simulink model "SF051A_SnsrOffsLrng"  (R2013b)
settings: Solver=FixedStepDiscrete  SolverMode=SingleTasking  StartTime=0.0  StopTime=1  FixedStep=0.002  RelTol=1e-3
undefined symbols (not defined in the file): ARCHGLBPRM_10MILLISEC_SEC_F32, ARCHGLBPRM_2MILLISEC_SEC_F32, ARCHGLBPRM_2PI_ULS_F32, ARCHGLBPRM_FLOATZEROTHD_ULS_F32, ARCHGLBPRM_PIOVER180_ULS_F32, CNV100MICROSECTOMILLISEC_MILLISECPERCNT_F32, CNV100MICROSECTOSEC_SECPERCNT_F32, COVRAMTRXNIT_ULS_F32, HWAUTHYTHD_ULS_F32, HWTQLRNGSTSLRND_CNT_U08, HWTQLRNGSTSNEGOFFS_CNT_U08, HWTQLRNGSTSNOTLRND_CNT_U08, HWTQLRNGSTSPOSOFFS_CNT_U08, HWTQLRNGSTSZEROOFFS_CNT_U08, HWTQLRNGTMRHILIM_SEC_F32, IDYMTRX_ULS_F32, IVS10MS_ULSPERSEC_F32, LRNGFILTICON_ULS_F32, NvmGetErrSts1, ONE_ULS_F32, SnsrOffsLrnd, SnsrOffsLrngFctEna, SnsrOffsLrngHwAgLrngDrvgDstThd, SnsrOffsLrngHwAgLrngEna, SnsrOffsLrngHwAgLrngHwVelThd, SnsrOffsLrngHwAgLrngSysTqThd, SnsrOffsLrngHwAgLrngSysTqThdMed, SnsrOffsLrngHwAgLrngSysTqThdTrustd, SnsrOffsLrngHwAgLrngSysTqThdWide, SnsrOffsLrngHwAgLrngTi, SnsrOffsLrngHwAgLrngVehSpdThd, SnsrOffsLrngHwAgLrngYawOffsDbnd, SnsrOffsLrngHwAgLrngYawRateThd, SnsrOffsLrngHwAgOffsLim, SnsrOffsLrngHwTqLrngEna, SnsrOffsLrngHwTqLrngEnaTiThd, SnsrOffsLrngHwTqLrngHwAgDbnd, SnsrOffsLrngHwTqLrngHwAgThd, SnsrOffsLrngHwTqLrngHwTqThd, SnsrOffsLrngHwTqLrngHwTqZeroOffsThd, SnsrOffsLrngHwTqLrngHwVelThd, SnsrOffsLrngHwTqLrngMeasTi, SnsrOffsLrngHwTqLrngMeasTiScar, SnsrOffsLrngHwTqLrngSampleImbThd1, SnsrOffsLrngHwTqLrngSampleImbThd2, SnsrOffsLrngHwTqLrngSampleThd1, SnsrOffsLrngHwTqLrngSampleThd2, SnsrOffsLrngHwTqLrngTiWghtCoeff, SnsrOffsLrngHwTqLrngVehSpdThd, SnsrOffsLrngHwTqOffsLim, SnsrOffsLrngSampleCntForHwTqLrngRst, SnsrOffsLrngTqInpDetnPwrEstimnThd, SnsrOffsLrngTqInpDetnSinGenrAmp, SnsrOffsLrngTqInpDetnSinGenrFrq, SnsrOffsLrngTqInpDetnStg1FilGain, SnsrOffsLrngTqInpDetnStg1WinSize, SnsrOffsLrngTqInpDetnStg2FilGainCen, SnsrOffsLrngTqInpDetnStg2FilGainDwn, SnsrOffsLrngTqInpDetnStg2FilGainUp, SnsrOffsLrngTqInpDetnStg2WinSize ... (+15)
libraries: Fil x34, FixdToFloat x17, FloatToFixd x16, NxtrLim x15, simulink x12, NxtrAbslt x12, NxtrNvM x8, NxtrMin x5, NxtrMath x3
(part 2 of 11)

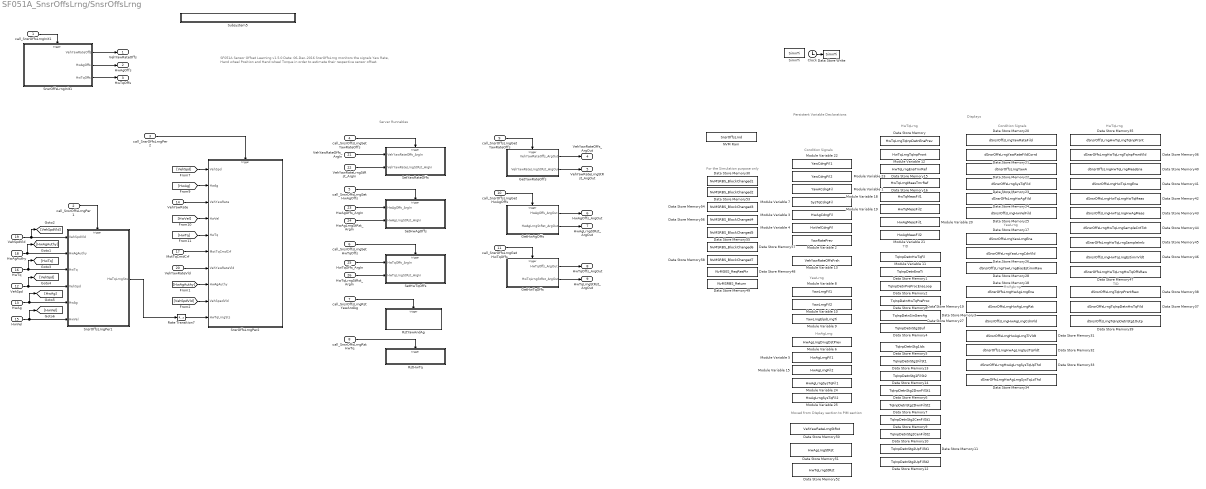
== system SF051A_SnsrOffsLrng/SnsrOffsLrng ==
  note: Moved from DIsplay section to PIM section
  note: For the Simulation purpose only
  note: TID
  note: TID
  note: Condition Signals
  note: Server Runnables
  note: Persistent Variable Declarations
  note: Displays
  note: YawLrng
  note: HwAgLrng
  note: HwTqLrng
  note: Condition Signals
  note: YawLrng
  note: HwAgLrng
  note: HwTqLrng
  note: SF051A  Sensor Offset Learning
      | v1.5.0 	Date: 06-Dec-2016
      |
      | SnsrOffsLrng monitors the signals Yaw Rate, Hand wheel Position and Hand wheel Torque in order to estimate their respective sensor offset.
  call_SnsrOffsLrngInit1 : Inport  RequirementInfo={'linktype_rmi_doors' '0000babd (/E-STEER Core/SubSystem Specifications/Application Functions/SF051A Sensor Offset Learning)' '#SF051A_46' 'true' 'REQ:SF051A_46' '' ; 'linktype_rmi_doors' '0000babd (/E-STEER Core/SubSystem Specifications/Application Functions/SF051A Sensor Offset Learning)' '#SF051A_210' 'true' 'REQ:SF051A_210' '' } %GIDa_b5548396_b826_4291_b305_596c7c623535
  call_SnsrOffsLrngPer1 : Inport  RequirementInfo={'linktype_rmi_doors' '0000babd (/E-STEER Core/SubSystem Specifications/Application Functions/SF051A Sensor Offset Learning)' '#SF051A_207' 'true' 'REQ:SF051A_207' '' } %GIDa_b76faf1e_0a38_4892_bc53_8cf50d1431b9  Port=2
  call_SnsrOffsLrngPer2 : Inport  RequirementInfo={'linktype_rmi_doors' '0000babd (/E-STEER Core/SubSystem Specifications/Application Functions/SF051A Sensor Offset Learning)' '#SF051A_206' 'true' 'REQ:SF051A_206' '' ; 'linktype_rmi_doors' '0000babd (/E-STEER Core/SubSystem Specifications/Application Functions/SF051A Sensor Offset Learning)' '#SF051A_208' 'true' 'REQ:SF051A_208' '' } %GIDa_53f91c8f_8084_4b7b_a29a_1f5e6264ef74  Port=3
  call_SnsrOffsLrngSetYawRateOffs : Inport  RequirementInfo={'linktype_rmi_doors' '0000babd (/E-STEER Core/SubSystem Specifications/Application Functions/SF051A Sensor Offset Learning)' '#SF051A_58' 'true' 'REQ:SF051A_58' '' ; 'linktype_rmi_doors' '0000babd (/E-STEER Core/SubSystem Specifications/Application Functions/SF051A Sensor Offset Learning)' '#SF051A_237' 'true' 'REQ:SF051A_237' '' } %GIDa_9ebfcf6d_e478_413c_8c0c_a98fbe6df9d3  Port=4
  call_SnsrOffsLrngSetHwAgOffs : Inport  RequirementInfo={'linktype_rmi_doors' '0000babd (/E-STEER Core/SubSystem Specifications/Application Functions/SF051A Sensor Offset Learning)' '#SF051A_215' 'true' 'REQ:SF051A_215' '' ; 'linktype_rmi_doors' '0000babd (/E-STEER Core/SubSystem Specifications/Application Functions/SF051A Sensor Offset Learning)' '#SF051A_236' 'true' 'REQ:SF051A_236' '' } %GIDa_c1056425_e33c_42d4_9d68_7c8d70d8efa0  Port=5
  call_SnsrOffsLrngSetHwTqOffs : Inport  RequirementInfo={'linktype_rmi_doors' '0000babd (/E-STEER Core/SubSystem Specifications/Application Functions/SF051A Sensor Offset Learning)' '#SF051A_213' 'true' 'REQ:SF051A_213' '' ; 'linktype_rmi_doors' '0000babd (/E-STEER Core/SubSystem Specifications/Application Functions/SF051A Sensor Offset Learning)' '#SF051A_238' 'true' 'REQ:SF051A_238' '' } %GIDa_875b11dc_9366_4bb8_a936_d7d6b5c30bfa  Port=6
  call_SnsrOffsLrngRstYawAndAg : Inport  RequirementInfo={'linktype_rmi_doors' '0000babd (/E-STEER Core/SubSystem Specifications/Application Functions/SF051A Sensor Offset Learning)' '#SF051A_211' 'true' 'REQ:SF051A_211' '' ; 'linktype_rmi_doors' '0000babd (/E-STEER Core/SubSystem Specifications/Application Functions/SF051A Sensor Offset Learning)' '#SF051A_234' 'true' 'REQ:SF051A_234' '' } %GIDa_4fb6cb0e_ae58_45eb_a23a_8ef4f0284ae6  Port=7
  call_SnsrOffsLrngRstHwTq : Inport  RequirementInfo={'linktype_rmi_doors' '0000babd (/E-STEER Core/SubSystem Specifications/Application Functions/SF051A Sensor Offset Learning)' '#SF051A_216' 'true' 'REQ:SF051A_216' '' ; 'linktype_rmi_doors' '0000babd (/E-STEER Core/SubSystem Specifications/Application Functions/SF051A Sensor Offset Learning)' '#SF051A_235' 'true' 'REQ:SF051A_235' '' } %GIDa_99803fa3_df4f_4cf4_914f_3ed5b7add009  Port=8
  call_SnsrOffsLrngGetYawRateOffs : Inport  RequirementInfo={'linktype_rmi_doors' '0000babd (/E-STEER Core/SubSystem Specifications/Application Functions/SF051A Sensor Offset Learning)' '#SF051A_217' 'true' 'REQ:SF051A_217' '' ; 'linktype_rmi_doors' '0000babd (/E-STEER Core/SubSystem Specifications/Application Functions/SF051A Sensor Offset Learning)' '#SF051A_229' 'true' 'REQ:SF051A_229' '' } %GIDa_2fe70a0d_0969_4657_91b9_882eb0d6e8f3  Port=9
  call_SnsrOffsLrngGetHwAgOffs : Inport  RequirementInfo={'linktype_rmi_doors' '0000babd (/E-STEER Core/SubSystem Specifications/Application Functions/SF051A Sensor Offset Learning)' '#SF051A_214' 'true' 'REQ:SF051A_214' '' ; 'linktype_rmi_doors' '0000babd (/E-STEER Core/SubSystem Specifications/Application Functions/SF051A Sensor Offset Learning)' '#SF051A_231' 'true' 'REQ:SF051A_231' '' } %GIDa_e15fe6be_8261_450e_92cb_69dfcf136740  Port=10
  call_SnsrOffsLrngGetHwTqOffs : Inport  RequirementInfo={'linktype_rmi_doors' '0000babd (/E-STEER Core/SubSystem Specifications/Application Functions/SF051A Sensor Offset Learning)' '#SF051A_212' 'true' 'REQ:SF051A_212' '' ; 'linktype_rmi_doors' '0000babd (/E-STEER Core/SubSystem Specifications/Application Functions/SF051A Sensor Offset Learning)' '#SF051A_233' 'true' 'REQ:SF051A_233' '' } %GIDa_11a16519_835e_433c_aee1_e13e931b852c  Port=11
  VehSpd : Inport  RequirementInfo={'linktype_rmi_doors' '0000babd (/E-STEER Core/SubSystem Specifications/Application Functions/SF051A Sensor Offset Learning)' '#SF051A_73' 'true' 'REQ:SF051A_73' '' } %GIDa_6cab4be4_5aaa_4f06_92e7_199f0ab886cf  Port=12
  HwAg : Inport  RequirementInfo={'linktype_rmi_doors' '0000babd (/E-STEER Core/SubSystem Specifications/Application Functions/SF051A Sensor Offset Learning)' '#SF051A_71' 'true' 'REQ:SF051A_71' '' } %GIDa_43d75a5a_0460_4bf8_8d04_3cab9ef42970  Port=13
  VehYawRate : Inport  RequirementInfo={'linktype_rmi_doors' '0000babd (/E-STEER Core/SubSystem Specifications/Application Functions/SF051A Sensor Offset Learning)' '#SF051A_74' 'true' 'REQ:SF051A_74' '' } %GIDa_85702be3_759d_431f_afdd_1834d4451958  Port=14
  HwVel : Inport  RequirementInfo={'linktype_rmi_doors' '0000babd (/E-STEER Core/SubSystem Specifications/Application Functions/SF051A Sensor Offset Learning)' '#SF051A_76' 'true' 'REQ:SF051A_76' '' } %GIDa_aea7e932_9aba_450e_a5e8_854429f45d9e  Port=15
  HwTq : Inport  RequirementInfo={'linktype_rmi_doors' '0000babd (/E-STEER Core/SubSystem Specifications/Application Functions/SF051A Sensor Offset Learning)' '#SF051A_12' 'true' 'REQ:SF051A_12' '' } %GIDa_419a1852_02b0_4166_858b_b9defd51bcfd  Port=16
  MotTqCmdCrf : Inport  RequirementInfo={'linktype_rmi_doors' '0000babd (/E-STEER Core/SubSystem Specifications/Application Functions/SF051A Sensor Offset Learning)' '#SF051A_78' 'true' 'REQ:SF051A_78' '' } %GIDa_8d4508d2_1c4e_4f52_beaa_b504c4c90863  Port=17
  HwAgAuthy : Inport  RequirementInfo={'linktype_rmi_doors' '0000babd (/E-STEER Core/SubSystem Specifications/Application Functions/SF051A Sensor Offset Learning)' '#SF051A_75' 'true' 'REQ:SF051A_75' '' } %GIDa_db428556_ad0a_4a7e_ac2f_05533f125a8d  Port=18
  VehSpdVld : Inport  RequirementInfo={'linktype_rmi_doors' '0000babd (/E-STEER Core/SubSystem Specifications/Application Functions/SF051A Sensor Offset Learning)' '#SF051A_72' 'true' 'REQ:SF051A_72' '' } %GIDa_549d97e8_51ee_4f7d_a4b4_1f4d4fa29ac3  Port=19
  VehYawRateVld : Inport  RequirementInfo={'linktype_rmi_doors' '0000babd (/E-STEER Core/SubSystem Specifications/Application Functions/SF051A Sensor Offset Learning)' '#SF051A_77' 'true' 'REQ:SF051A_77' '' } %GIDa_9dcd395b_e912_4846_98d8_9746842c61cb  Port=20
  VehYawRateOffs_ArgIn : Inport  RequirementInfo={'linktype_rmi_doors' '0000babd (/E-STEER Core/SubSystem Specifications/Application Functions/SF051A Sensor Offset Learning)' '#SF051A_58' 'true' 'REQ:SF051A_58' '' } %GIDa_f87127ae_4fd6_4799_a67b_96b70cf59f57  Port=21
  VehYawRateLrngStRst_ArgIn : Inport  RequirementInfo={'linktype_rmi_doors' '0000babd (/E-STEER Core/SubSystem Specifications/Application Functions/SF051A Sensor Offset Learning)' '#SF051A_237' 'true' 'REQ:SF051A_237' '' } %GIDa_de74ad38_9d1d_42b4_98c9_5d5518144ab9  Port=22
  HwAgOffs_ArgIn : Inport  RequirementInfo={'linktype_rmi_doors' '0000babd (/E-STEER Core/SubSystem Specifications/Application Functions/SF051A Sensor Offset Learning)' '#SF051A_215' 'true' 'REQ:SF051A_215' '' } %GIDa_6970447d_a6e4_4a38_8aa3_8925f782d5d0  Port=23
  HwAgLrngStRst_ArgIn : Inport  RequirementInfo={'linktype_rmi_doors' '0000babd (/E-STEER Core/SubSystem Specifications/Application Functions/SF051A Sensor Offset Learning)' '#SF051A_236' 'true' 'REQ:SF051A_236' '' } %GIDa_7c9b4228_d04e_41fe_8d4c_bf60f37f9eec  Port=24
  HwTqOffs_ArgIn : Inport  RequirementInfo={'linktype_rmi_doors' '0000babd (/E-STEER Core/SubSystem Specifications/Application Functions/SF051A Sensor Offset Learning)' '#SF051A_213' 'true' 'REQ:SF051A_213' '' } %GIDa_303f314c_88b6_4fa0_bca5_4af63bedbea5  Port=25
  HwTqLrngStRst_ArgIn : Inport  RequirementInfo={'linktype_rmi_doors' '0000babd (/E-STEER Core/SubSystem Specifications/Application Functions/SF051A Sensor Offset Learning)' '#SF051A_238' 'true' 'REQ:SF051A_238' '' } %GIDa_34ca438f_6084_484d_a532_1ca155d267e9  Port=26
  Clock : Clock
  Data Store Memory : DataStoreMemory  DataStoreName=HwTqLrngTqInpDetnEnaPrev  OutDataTypeStr=boolean  StateMustResolveToSignalObject=on
  Data Store Memory1 : DataStoreMemory  DataStoreName=TqInpDetnEnaTi  StateMustResolveToSignalObject=on
  Data Store Memory10 : DataStoreMemory  DataStoreName=TqInpDetnStg2CenFilSt2  StateMustResolveToSignalObject=on
  Data Store Memory11 : DataStoreMemory  DataStoreName=TqInpDetnStg2UpFilSt1  StateMustResolveToSignalObject=on
  Data Store Memory12 : DataStoreMemory  DataStoreName=TqInpDetnStg2UpFilSt2  StateMustResolveToSignalObject=on
  Data Store Memory13 : DataStoreMemory  DataStoreName=TqInpDetnStg1FilSt1  StateMustResolveToSignalObject=on
  Data Store Memory14 : DataStoreMemory  DataStoreName=TqInpDetnStg1FilSt2  StateMustResolveToSignalObject=on
  Data Store Memory15 : DataStoreMemory  DataStoreName=HwTqLrngEnaTmrRef  StateMustResolveToSignalObject=on
  Data Store Memory16 : DataStoreMemory  DataStoreName=HwTqLrngMeasTmrRef  OutDataTypeStr=uint32  StateMustResolveToSignalObject=on
  Data Store Memory17 : DataStoreMemory  DataStoreName=dSnsrOffsLrngYawLrngEna  StateMustResolveToSignalObject=on
  Data Store Memory18 : DataStoreMemory  DataStoreName=dSnsrOffsLrngHwAgLrngEna  StateMustResolveToSignalObject=on
  Data Store Memory19 : DataStoreMemory  DataStoreName=dSnsrOffsLrngHwAgLrngRst  StateMustResolveToSignalObject=on
  Data Store Memory2 : DataStoreMemory  DataStoreName=TqInpDetnPreProcEnaLoop  OutDataTypeStr=uint16  StateMustResolveToSignalObject=on
  Data Store Memory20 : DataStoreMemory  DataStoreName=dSnsrOffsLrngYawRateFild  StateMustResolveToSignalObject=on
  Data Store Memory21 : DataStoreMemory  DataStoreName=dSnsrOffsLrngYawRateFildCorrd  StateMustResolveToSignalObject=on
  Data Store Memory22 : DataStoreMemory  DataStoreName=dSnsrOffsLrngYawA  StateMustResolveToSignalObject=on
  Data Store Memory23 : DataStoreMemory  DataStoreName=dSnsrOffsLrngSysTqFild  StateMustResolveToSignalObject=on
  Data Store Memory24 : DataStoreMemory  DataStoreName=dSnsrOffsLrngHwAgFild  StateMustResolveToSignalObject=on
  Data Store Memory25 : DataStoreMemory  DataStoreName=dSnsrOffsLrngHwVelFild  StateMustResolveToSignalObject=on
  Data Store Memory26 : DataStoreMemory  DataStoreName=dSnsrOffsLrngYawLrngCdnVld  StateMustResolveToSignalObject=on
  Data Store Memory27 : DataStoreMemory  DataStoreName=dSnsrOffsLrngHwAgLrngCdnVld  StateMustResolveToSignalObject=on
  Data Store Memory28 : DataStoreMemory  DataStoreName=dSnsrOffsLrngYawLrngBiasEstimnRaw  StateMustResolveToSignalObject=on
  Data Store Memory3 : DataStoreMemory  DataStoreName=TqInpDetnSinGenrAg  StateMustResolveToSignalObject=on
  Data Store Memory30 : DataStoreMemory  DataStoreName=NvMSRBS_BlockChanged1
  Data Store Memory31 : DataStoreMemory  DataStoreName=dSnsrOffsLrngHwAgLrngTiVldt  StateMustResolveToSignalObject=on
  Data Store Memory32 : DataStoreMemory  DataStoreName=dSnsrOffsLrngHwAgLrngSysTqVldt  StateMustResolveToSignalObject=on
  Data Store Memory33 : DataStoreMemory  DataStoreName=dSnsrOffsLrngHwAgLrngSysTqUpThd  StateMustResolveToSignalObject=on
  Data Store Memory34 : DataStoreMemory  DataStoreName=dSnsrOffsLrngHwAgLrngSysTqLoThd  StateMustResolveToSignalObject=on
  Data Store Memory35 : DataStoreMemory  DataStoreName=dSnsrOffsLrngHwTqLrngTqInpPrsnt  StateMustResolveToSignalObject=on
  Data Store Memory36 : DataStoreMemory  DataStoreName=dSnsrOffsLrngHwTqLrngTqInpPrsntVld  StateMustResolveToSignalObject=on
  Data Store Memory37 : DataStoreMemory  DataStoreName=dSnsrOffsLrngTqInpDetnHwTqFild  StateMustResolveToSignalObject=on
  Data Store Memory38 : DataStoreMemory  DataStoreName=dSnsrOffsLrngTqInpPrsntRaw  StateMustResolveToSignalObject=on
  Data Store Memory39 : DataStoreMemory  DataStoreName=dSnsrOffsLrngTqInpDetnStg1Outp  StateMustResolveToSignalObject=on
  Data Store Memory4 : DataStoreMemory  DataStoreName=TqInpDetnStg1Buf  InitialValue=[]  StateMustResolveToSignalObject=on
      settings: AttributesFormatString=Initialize as array of 72 zeros because buffer size cal = 1 to 72.
  Data Store Memory40 : DataStoreMemory  DataStoreName=dSnsrOffsLrngHwTqLrngMeasEna  StateMustResolveToSignalObject=on
  Data Store Memory41 : DataStoreMemory  DataStoreName=dSnsrOffsLrngHwTqLrngEna  StateMustResolveToSignalObject=on
  Data Store Memory42 : DataStoreMemory  DataStoreName=dSnsrOffsLrngHwTqLrngHwTqMeas  StateMustResolveToSignalObject=on
  Data Store Memory43 : DataStoreMemory  DataStoreName=dSnsrOffsLrngHwTqLrngHwAgMeas  StateMustResolveToSignalObject=on
  Data Store Memory44 : DataStoreMemory  DataStoreName=dSnsrOffsLrngHwTqLrngSampleCntTot  StateMustResolveToSignalObject=on
  Data Store Memory45 : DataStoreMemory  DataStoreName=dSnsrOffsLrngHwTqLrngSampleImb  StateMustResolveToSignalObject=on
  Data Store Memory46 : DataStoreMemory  DataStoreName=dSnsrOffsLrngHwTqLrngEstimnVldt  StateMustResolveToSignalObject=on
  Data Store Memory47 : DataStoreMemory  DataStoreName=dSnsrOffsLrngHwTqLrngHwTqOffsRaw  StateMustResolveToSignalObject=on
  Data Store Memory48 : DataStoreMemory  DataStoreName=NvMGES_ReqResPtr  InitialValue=NvmGetErrSts1.REQUEST_NOT_OK  OutDataTypeStr=Enum: NvmGetErrSts1
  Data Store Memory49 : DataStoreMemory  DataStoreName=NvMSRBS_Return
  Data Store Memory5 : DataStoreMemory  DataStoreName=TqInpDetnStg1Idx  StateMustResolveToSignalObject=on
  Data Store Memory50 : DataStoreMemory  DataStoreName=VehYawRateLrngStRst  StateMustResolveToSignalObject=on
  Data Store Memory51 : DataStoreMemory  DataStoreName=HwAgLrngStRst  StateMustResolveToSignalObject=on
  Data Store Memory52 : DataStoreMemory  DataStoreName=HwTqLrngStRst  StateMustResolveToSignalObject=on
  Data Store Memory53 : DataStoreMemory  DataStoreName=NvMSRBS_BlockChanged2
  Data Store Memory54 : DataStoreMemory  DataStoreName=NvMSRBS_BlockChanged3
  Data Store Memory55 : DataStoreMemory  DataStoreName=NvMSRBS_BlockChanged5
  Data Store Memory56 : DataStoreMemory  DataStoreName=NvMSRBS_BlockChanged4
  Data Store Memory57 : DataStoreMemory  DataStoreName=NvMSRBS_BlockChanged6
  Data Store Memory58 : DataStoreMemory  DataStoreName=NvMSRBS_BlockChanged7
  Data Store Memory6 : DataStoreMemory  DataStoreName=TqInpDetnStg2DwnFilSt1  StateMustResolveToSignalObject=on
  Data Store Memory7 : DataStoreMemory  DataStoreName=TqInpDetnStg2DwnFilSt2  StateMustResolveToSignalObject=on
  Data Store Memory8 : DataStoreMemory  DataStoreName=TqInpDetnHwTqPreProc  StateMustResolveToSignalObject=on
  Data Store Memory9 : DataStoreMemory  DataStoreName=TqInpDetnStg2CenFilSt1  StateMustResolveToSignalObject=on
  Data Store Write : DataStoreWrite  DataStoreName=SimnTi
  GetHwAgOffs : Subsystem  RequirementInfo={'linktype_rmi_doors' '0000babd (/E-STEER Core/SubSystem Specifications/Application Functions/SF051A Sensor Offset Learning)' '#SF051A_214' 'true' 'REQ:SF051A_214' '' ; 'linktype_rmi_doors' '0000babd (/E-STEER Core/SubSystem Specifications/Application Functions/SF051A Sensor Offset Learning)' '#SF051A_231' 'true' 'REQ:SF051A_231' '' } %GIDa_829ee463_2f90_4434_8814_18ee114c17a8  TreatAsAtomicUnit=on
  GetHwTqOffs : Subsystem  RequirementInfo={'linktype_rmi_doors' '0000babd (/E-STEER Core/SubSystem Specifications/Application Functions/SF051A Sensor Offset Learning)' '#SF051A_212' 'true' 'REQ:SF051A_212' '' ; 'linktype_rmi_doors' '0000babd (/E-STEER Core/SubSystem Specifications/Application Functions/SF051A Sensor Offset Learning)' '#SF051A_233' 'true' 'REQ:SF051A_233' '' } %GIDa_f3af8530_8b46_4cec_b6bb_ea1c7cec3483  TreatAsAtomicUnit=on
  GetYawRateOffs : Subsystem  RequirementInfo={'linktype_rmi_doors' '0000babd (/E-STEER Core/SubSystem Specifications/Application Functions/SF051A Sensor Offset Learning)' '#SF051A_217' 'true' 'REQ:SF051A_217' '' ; 'linktype_rmi_doors' '0000babd (/E-STEER Core/SubSystem Specifications/Application Functions/SF051A Sensor Offset Learning)' '#SF051A_229' 'true' 'REQ:SF051A_229' '' } %GIDa_bc715bf0_598f_44bb_a83a_ee16c1cb044c  TreatAsAtomicUnit=on
  Module Variable 1 : DataStoreMemory  DataStoreName=YawACdngFil  InitialValue=struct('FilSt',single(0),'FilGain',single(0))  StateMustResolveToSignalObject=on
  Module Variable 10 : DataStoreMemory  DataStoreName=YawLrngFil2  InitialValue=struct('FilSt',single(0),'FilGain',single(0))  StateMustResolveToSignalObject=on
  Module Variable 11 : DataStoreMemory  DataStoreName=TqInpDetnHwTqFil  InitialValue=struct('FilSt',single(0),'FilGain',single(0))  StateMustResolveToSignalObject=on
  Module Variable 12 : DataStoreMemory  DataStoreName=HwTqLrngTqInpPrsnt  OutDataTypeStr=boolean  StateMustResolveToSignalObject=on
  Module Variable 13 : DataStoreMemory  DataStoreName=VehYawRateOffsFrsh  StateMustResolveToSignalObject=on
  Module Variable 15 : DataStoreMemory  DataStoreName=HwAgLrngFil2  InitialValue=struct('FilSt',single(0),'FilGain',single(0))  StateMustResolveToSignalObject=on
  Module Variable 18 : DataStoreMemory  DataStoreName=HwTqMeasFil1  InitialValue=struct('FilSt',single(0),'FilGain',single(0))  StateMustResolveToSignalObject=on
  Module Variable 19 : DataStoreMemory  DataStoreName=HwTqMeasFil2  InitialValue=struct('FilSt',single(0),'FilGain',single(0))  StateMustResolveToSignalObject=on
  Module Variable 2 : DataStoreMemory  DataStoreName=YawRatePrev  StateMustResolveToSignalObject=on
  Module Variable 20 : DataStoreMemory  DataStoreName=HwAgMeasFil1  InitialValue=struct('FilSt',single(0),'FilGain',single(0))  StateMustResolveToSignalObject=on
  Module Variable 21 : DataStoreMemory  DataStoreName=HwAgMeasFil2  InitialValue=struct('FilSt',single(0),'FilGain',single(0))  StateMustResolveToSignalObject=on
  Module Variable 22 : DataStoreMemory  DataStoreName=YawCdngFil1  InitialValue=struct('FilSt',single(0),'FilGain',single(0))  StateMustResolveToSignalObject=on
  Module Variable 23 : DataStoreMemory  DataStoreName=YawCdngFil2  InitialValue=struct('FilSt',single(0),'FilGain',single(0))  StateMustResolveToSignalObject=on
  Module Variable 24 : DataStoreMemory  DataStoreName=HwAgLrngSysTqFil1  InitialValue=struct('FilSt',single(0),'FilGain',single(0))  StateMustResolveToSignalObject=on
  Module Variable 25 : DataStoreMemory  DataStoreName=HwAgLrngSysTqFil2  InitialValue=struct('FilSt',single(0),'FilGain',single(0))  StateMustResolveToSignalObject=on
  Module Variable 3 : DataStoreMemory  DataStoreName=HwAgCdngFil  InitialValue=struct('FilSt',single(0),'FilGain',single(0))  StateMustResolveToSignalObject=on
  Module Variable 4 : DataStoreMemory  DataStoreName=HwVelCdngFil  InitialValue=struct('FilSt',single(0),'FilGain',single(0))  StateMustResolveToSignalObject=on
  Module Variable 5 : DataStoreMemory  DataStoreName=HwAgLrngFil1  InitialValue=struct('FilSt',single(0),'FilGain',single(0))  StateMustResolveToSignalObject=on
  Module Variable 6 : DataStoreMemory  DataStoreName=HwAgLrngDrvgDstPrev  OutDataTypeStr=single  StateMustResolveToSignalObject=on
  Module Variable 7 : DataStoreMemory  DataStoreName=SysTqCdngFil  InitialValue=struct('FilSt',single(0),'FilGain',single(0))  StateMustResolveToSignalObject=on
  Module Variable 8 : DataStoreMemory  DataStoreName=YawLrngFil1  InitialValue=struct('FilSt',single(0),'FilGain',single(0))  StateMustResolveToSignalObject=on
  Module Variable 9 : DataStoreMemory  DataStoreName=YawLrngElpdLrngTi  StateMustResolveToSignalObject=on
  NVM Ram : DataStoreMemory  DataStoreName=SnsrOffsLrnd  InitialValue=[]  OutDataTypeStr=Bus: SnsrLrndOffsRec2  StateMustResolveToSignalObject=on
  Rate Transition7 : RateTransition
  RstHwTq : Subsystem  RequirementInfo={'linktype_rmi_doors' '0000babd (/E-STEER Core/SubSystem Specifications/Application Functions/SF051A Sensor Offset Learning)' '#SF051A_216' 'true' 'REQ:SF051A_216' '' ; 'linktype_rmi_doors' '0000babd (/E-STEER Core/SubSystem Specifications/Application Functions/SF051A Sensor Offset Learning)' '#SF051A_235' 'true' 'REQ:SF051A_235' '' } %GIDa_35cf7fbd_44fa_44c1_a04c_61a9eb1f15ad  TreatAsAtomicUnit=on
  RstYawAndAg : Subsystem  RequirementInfo={'linktype_rmi_doors' '0000babd (/E-STEER Core/SubSystem Specifications/Application Functions/SF051A Sensor Offset Learning)' '#SF051A_211' 'true' 'REQ:SF051A_211' '' ; 'linktype_rmi_doors' '0000babd (/E-STEER Core/SubSystem Specifications/Application Functions/SF051A Sensor Offset Learning)' '#SF051A_234' 'true' 'REQ:SF051A_234' '' } %GIDa_11c25bcd_c482_473a_959d_e87e5242baa8  TreatAsAtomicUnit=on
  SetHwAgOffs : Subsystem  RequirementInfo={'linktype_rmi_doors' '0000babd (/E-STEER Core/SubSystem Specifications/Application Functions/SF051A Sensor Offset Learning)' '#SF051A_215' 'true' 'REQ:SF051A_215' '' ; 'linktype_rmi_doors' '0000babd (/E-STEER Core/SubSystem Specifications/Application Functions/SF051A Sensor Offset Learning)' '#SF051A_236' 'true' 'REQ:SF051A_236' '' } %GIDa_5e7add5c_5e74_41c4_b4e3_9ae8ec34988d  TreatAsAtomicUnit=on
  SetHwTqOffs : Subsystem  RequirementInfo={'linktype_rmi_doors' '0000babd (/E-STEER Core/SubSystem Specifications/Application Functions/SF051A Sensor Offset Learning)' '#SF051A_213' 'true' 'REQ:SF051A_213' '' ; 'linktype_rmi_doors' '0000babd (/E-STEER Core/SubSystem Specifications/Application Functions/SF051A Sensor Offset Learning)' '#SF051A_238' 'true' 'REQ:SF051A_238' '' } %GIDa_674f277a_5ffd_42ee_acb4_132d2bed9af9  TreatAsAtomicUnit=on
  SetYawRateOffs : Subsystem  RequirementInfo={'linktype_rmi_doors' '0000babd (/E-STEER Core/SubSystem Specifications/Application Functions/SF051A Sensor Offset Learning)' '#SF051A_58' 'true' 'REQ:SF051A_58' '' ; 'linktype_rmi_doors' '0000babd (/E-STEER Core/SubSystem Specifications/Application Functions/SF051A Sensor Offset Learning)' '#SF051A_237' 'true' 'REQ:SF051A_237' '' } %GIDa_03f3f985_4ced_42ce_b677_aa375563c351  TreatAsAtomicUnit=on
  SimnTi : DataStoreMemory  DataStoreName=SimnTi
  SnsrOffsLrngInit1 : Subsystem  RequirementInfo={'linktype_rmi_doors' '0000babd (/E-STEER Core/SubSystem Specifications/Application Functions/SF051A Sensor Offset Learning)' '#SF051A_46' 'true' 'REQ:SF051A_46' '' ; 'linktype_rmi_doors' '0000babd (/E-STEER Core/SubSystem Specifications/Application Functions/SF051A Sensor Offset Learning)' '#SF051A_210' 'true' 'REQ:SF051A_210' '' } %GIDa_e5526f40_69ec_41c8_aeb3_272a8ad562fe  TreatAsAtomicUnit=on
  SnsrOffsLrngPer1 : Subsystem  RequirementInfo={'linktype_rmi_doors' '0000babd (/E-STEER Core/SubSystem Specifications/Application Functions/SF051A Sensor Offset Learning)' '#SF051A_207' 'true' 'REQ:SF051A_207' '' ; 'linktype_rmi_doors' '0000babd (/E-STEER Core/SubSystem Specifications/Application Functions/SF051A Sensor Offset Learning)' '#SF051A_150' 'true' 'REQ:SF051A_150' '' } %GIDa_18fd47b5_e5b3_49e8_b2eb_462539bdbc07  TreatAsAtomicUnit=on
  SnsrOffsLrngPer2 : Subsystem  RequirementInfo={'linktype_rmi_doors' '0000babd (/E-STEER Core/SubSystem Specifications/Application Functions/SF051A Sensor Offset Learning)' '#SF051A_206' 'true' 'REQ:SF051A_206' '' ; 'linktype_rmi_doors' '0000babd (/E-STEER Core/SubSystem Specifications/Application Functions/SF051A Sensor Offset Learning)' '#SF051A_208' 'true' 'REQ:SF051A_208' '' } %GIDa_9ad6eb25_dbe1_4fbc_8267_4845d305b716  TreatAsAtomicUnit=on
  Subsystem5 : Subsystem  Description=|  mask(Copyright Information){none=on}
      | Copyright info block.                                               
      |                                                                     
      | Place copyright information at the top of every subsystem in design.
      mask prompts: none "No parameters"
      mask help: Place copyright information at the top of every subsystem in design.
      mask Display:
      | NxtrConf = 'Nexteer Confidential';
      | 
      | sys = bdroot; %handle for the current model ("system")
      | first = get_param(sys,'Created');
      | first = first(end-3:end);  %year is last four digits
      | 
      | last = get_param(sys,'LastModifiedDate');
      | if isempty(last)
      |     last = datestr(now,'yyyy');
      | else
      |     last = last(end-3:end);
      | end
      | 
      | if strcmp(first,last)
      |     fprintf('%s -- Copyright %s Nexteer',NxtrConf,first)
      | else
      |     fprintf('%s -- %s%s- %s Nexteer',NxtrConf,char(169),first,last)
      | end
  VehYawRateOffs : Outport  RequirementInfo={'linktype_rmi_doors' '0000babd (/E-STEER Core/SubSystem Specifications/Application Functions/SF051A Sensor Offset Learning)' '#SF051A_79' 'true' 'REQ:SF051A_79' '' } %GIDa_74b7b237_2feb_4640_89f6_7308166d4c38
  HwAgOffs : Outport  RequirementInfo={'linktype_rmi_doors' '0000babd (/E-STEER Core/SubSystem Specifications/Application Functions/SF051A Sensor Offset Learning)' '#SF051A_80' 'true' 'REQ:SF051A_80' '' } %GIDa_6999a579_6919_44b1_9a7c_558ed8ee9dd3  Port=2
  HwTqOffs : Outport  RequirementInfo={'linktype_rmi_doors' '0000babd (/E-STEER Core/SubSystem Specifications/Application Functions/SF051A Sensor Offset Learning)' '#SF051A_16' 'true' 'REQ:SF051A_16' '' } %GIDa_7ed9d0c4_c855_44d3_9481_9311f85f734c  Port=3
  VehYawRateOffs_ArgOut : Outport  RequirementInfo={'linktype_rmi_doors' '0000babd (/E-STEER Core/SubSystem Specifications/Application Functions/SF051A Sensor Offset Learning)' '#SF051A_217' 'true' 'REQ:SF051A_217' '' } %GIDa_ed4643bf_f320_4bca_ad53_8d62e934aa82  Port=4
  VehYawRateLrngStRst_ArgOut : Outport  RequirementInfo={'linktype_rmi_doors' '0000babd (/E-STEER Core/SubSystem Specifications/Application Functions/SF051A Sensor Offset Learning)' '#SF051A_229' 'true' 'REQ:SF051A_229' '' } %GIDa_5454e49f_d2f7_4039_87a0_3c1a65138a11  Port=5
  HwAgOffs_ArgOut : Outport  RequirementInfo={'linktype_rmi_doors' '0000babd (/E-STEER Core/SubSystem Specifications/Application Functions/SF051A Sensor Offset Learning)' '#SF051A_214' 'true' 'REQ:SF051A_214' '' } %GIDa_d0957068_92dc_4fc8_a891_84ba21659084  Port=6
  HwAgLrngStRst_ArgOut : Outport  RequirementInfo={'linktype_rmi_doors' '0000babd (/E-STEER Core/SubSystem Specifications/Application Functions/SF051A Sensor Offset Learning)' '#SF051A_231' 'true' 'REQ:SF051A_231' '' } %GIDa_07ead7ae_0255_4448_9d02_649f17678103  Port=7
  HwTqOffs_ArgOut : Outport  RequirementInfo={'linktype_rmi_doors' '0000babd (/E-STEER Core/SubSystem Specifications/Application Functions/SF051A Sensor Offset Learning)' '#SF051A_212' 'true' 'REQ:SF051A_212' '' } %GIDa_1dddb811_c09d_4678_9846_2c2880d0f6fa  Port=8
  HwTqLrngStRst_ArgOut : Outport  RequirementInfo={'linktype_rmi_doors' '0000babd (/E-STEER Core/SubSystem Specifications/Application Functions/SF051A Sensor Offset Learning)' '#SF051A_233' 'true' 'REQ:SF051A_233' '' } %GIDa_e27f45cc_dae8_42b9_bd97_11f1d18acfdc  Port=9
  wires:
  call_SnsrOffsLrngPer2/1 -> SnsrOffsLrngPer2/Trigger
  SnsrOffsLrngInit1/1(VehYawRateOffs) -> VehYawRateOffs/1
  call_SnsrOffsLrngInit1/1 -> SnsrOffsLrngInit1/Trigger
  call_SnsrOffsLrngSetYawRateOffs/1 -> SetYawRateOffs/Trigger
  VehYawRateOffs_ArgIn/1 -> SetYawRateOffs/1(VehYawRateOffs_ArgIn)
  call_SnsrOffsLrngSetHwAgOffs/1 -> SetHwAgOffs/Trigger
  HwAgOffs_ArgIn/1 -> SetHwAgOffs/1(HwAgOffs_ArgIn)
  call_SnsrOffsLrngSetHwTqOffs/1 -> SetHwTqOffs/Trigger
  HwTqOffs_ArgIn/1 -> SetHwTqOffs/1(HwTqOffs_ArgIn)
  call_SnsrOffsLrngRstYawAndAg/1 -> RstYawAndAg/Trigger
  call_SnsrOffsLrngPer1/1 -> SnsrOffsLrngPer1/Trigger
  SnsrOffsLrngInit1/2(HwAgOffs) -> HwAgOffs/1
  SnsrOffsLrngInit1/3(HwTqOffs) -> HwTqOffs/1
  VehYawRateLrngStRst_ArgIn/1 -> SetYawRateOffs/2(VehYawRateLrngStRst_ArgIn)
  HwAgLrngStRst_ArgIn/1 -> SetHwAgOffs/2(HwAgLrngStRst_ArgIn)
  HwTqLrngStRst_ArgIn/1 -> SetHwTqOffs/2(HwTqLrngStRst_ArgIn)
  call_SnsrOffsLrngRstHwTq/1 -> RstHwTq/Trigger
  SnsrOffsLrngPer1/1(HwTqLrngSts) -> Rate Transition7/1
  VehSpdVld/1 -> [VehSpdVld], SnsrOffsLrngPer1/1(VehSpdVld)
  HwAgAuthy/1 -> SnsrOffsLrngPer1/2(HwAgAuthy), [HwAgAuthy]
  HwTq/1 -> SnsrOffsLrngPer1/3(HwTq), [HwTq]
  [HwAg] -> SnsrOffsLrngPer2/2(HwAg)
  VehYawRate/1 -> SnsrOffsLrngPer2/3(VehYawRate)
  [HwVel] -> SnsrOffsLrngPer2/4(HwVel)
  [HwTq] -> SnsrOffsLrngPer2/5(HwTq)
  MotTqCmdCrf/1 -> SnsrOffsLrngPer2/6(MotTqCmdCrf)
  VehYawRateVld/1 -> SnsrOffsLrngPer2/7(VehYawRateVld)
  [HwAgAuthy] -> SnsrOffsLrngPer2/8(HwAgAuthy)
  [VehSpdVld] -> SnsrOffsLrngPer2/9(VehSpedVld)
  Rate Transition7/1 -> SnsrOffsLrngPer2/10(HwTqLrngSts)
  Clock/1 -> Data Store Write/1
  HwVel/1 -> [HwVel], SnsrOffsLrngPer1/6(HwVel)
  HwAg/1 -> [HwAg], SnsrOffsLrngPer1/5(HwAg)
  VehSpd/1 -> [VehSpd], SnsrOffsLrngPer1/4(VehSpd)
  [VehSpd] -> SnsrOffsLrngPer2/1(VehSpd)
  call_SnsrOffsLrngGetYawRateOffs/1 -> GetYawRateOffs/Trigger
  GetYawRateOffs/1(VehYawRateOffs_ArgOut) -> VehYawRateOffs_ArgOut/1
  call_SnsrOffsLrngGetHwAgOffs/1 -> GetHwAgOffs/Trigger
  GetHwAgOffs/1(HwAgOffs_ArgOut) -> HwAgOffs_ArgOut/1
  call_SnsrOffsLrngGetHwTqOffs/1 -> GetHwTqOffs/Trigger
  GetHwTqOffs/1(HwTqOffs_ArgOut) -> HwTqOffs_ArgOut/1
  GetYawRateOffs/2(VehYawRateLrngStRst_ArgOut) -> VehYawRateLrngStRst_ArgOut/1
  GetHwAgOffs/2(HwAgLrngStRst_ArgOut) -> HwAgLrngStRst_ArgOut/1
  GetHwTqOffs/2(HwTqLrngStRst_ArgOut) -> HwTqLrngStRst_ArgOut/1

== system SF051A_SnsrOffsLrng/Subsystem5 ==

== system SF051A_SnsrOffsLrng/call_SnsrOffsLrngInit1 ==
  Enable : EnablePort
  FunctionCalGenerator : simulink/Ports & Subsystems/Function-Call Generator  sample_time=0  numberOfIterations=1
  Subsystem5 : Subsystem  Description=|  mask(Copyright Information){none=on}
      | Copyright info block.                                               
      |                                                                     
      | Place copyright information at the top of every subsystem in design.
      mask prompts: none "No parameters"
      mask help: Place copyright information at the top of every subsystem in design.
      mask Display:
      | NxtrConf = 'Nexteer Confidential';
      | 
      | sys = bdroot; %handle for the current model ("system")
      | first = get_param(sys,'Created');
      | first = first(end-3:end);  %year is last four digits
      | 
      | last = get_param(sys,'LastModifiedDate');
      | if isempty(last)
      |     last = datestr(now,'yyyy');
      | else
      |     last = last(end-3:end);
      | end
      | 
      | if strcmp(first,last)
      |     fprintf('%s -- Copyright %s Nexteer',NxtrConf,first)
      | else
      |     fprintf('%s -- %s%s- %s Nexteer',NxtrConf,char(169),first,last)
      | end
  call_SnsrOffsLrngInit1 : Outport
  wires:
  FunctionCalGenerator/1 -> call_SnsrOffsLrngInit1/1

== system SF051A_SnsrOffsLrng/call_SnsrOffsLrngPer1 ==
  Enable : EnablePort
  FunctionCalGenerator1 : simulink/Ports & Subsystems/Function-Call Generator  sample_time=.002  numberOfIterations=1
      settings: AttributesFormatString=%<sample_time> sec
  Subsystem5 : Subsystem  Description=|  mask(Copyright Information){none=on}
      | Copyright info block.                                               
      |                                                                     
      | Place copyright information at the top of every subsystem in design.
      mask prompts: none "No parameters"
      mask help: Place copyright information at the top of every subsystem in design.
      mask Display:
      | NxtrConf = 'Nexteer Confidential';
      | 
      | sys = bdroot; %handle for the current model ("system")
      | first = get_param(sys,'Created');
      | first = first(end-3:end);  %year is last four digits
      | 
      | last = get_param(sys,'LastModifiedDate');
      | if isempty(last)
      |     last = datestr(now,'yyyy');
      | else
      |     last = last(end-3:end);
      | end
      | 
      | if strcmp(first,last)
      |     fprintf('%s -- Copyright %s Nexteer',NxtrConf,first)
      | else
      |     fprintf('%s -- %s%s- %s Nexteer',NxtrConf,char(169),first,last)
      | end
  call_SnsrOffsLrngPer1 : Outport
  wires:
  FunctionCalGenerator1/1 -> call_SnsrOffsLrngPer1/1

== system SF051A_SnsrOffsLrng/call_SnsrOffsLrngPer2 ==
  Enable : EnablePort
  FunctionCallGenerator1 : simulink/Ports & Subsystems/Function-Call Generator  sample_time=.010  numberOfIterations=1
      settings: AttributesFormatString=%<sample_time> sec
  Subsystem5 : Subsystem  Description=|  mask(Copyright Information){none=on}
      | Copyright info block.                                               
      |                                                                     
      | Place copyright information at the top of every subsystem in design.
      mask prompts: none "No parameters"
      mask help: Place copyright information at the top of every subsystem in design.
      mask Display:
      | NxtrConf = 'Nexteer Confidential';
      | 
      | sys = bdroot; %handle for the current model ("system")
      | first = get_param(sys,'Created');
      | first = first(end-3:end);  %year is last four digits
      | 
      | last = get_param(sys,'LastModifiedDate');
      | if isempty(last)
      |     last = datestr(now,'yyyy');
      | else
      |     last = last(end-3:end);
      | end
      | 
      | if strcmp(first,last)
      |     fprintf('%s -- Copyright %s Nexteer',NxtrConf,first)
      | else
      |     fprintf('%s -- %s%s- %s Nexteer',NxtrConf,char(169),first,last)
      | end
  call_SnsrOffsLrngPer2 : Outport
  wires:
  FunctionCallGenerator1/1 -> call_SnsrOffsLrngPer2/1

== system SF051A_SnsrOffsLrng/ call_SnsrOffsLrngGetHwAgOffs/Subsystem5 ==

== system SF051A_SnsrOffsLrng/ call_SnsrOffsLrngGetHwTqOffs/Subsystem5 ==

== system SF051A_SnsrOffsLrng/ call_SnsrOffsLrngGetYawRateOffs/Subsystem5 ==

== system SF051A_SnsrOffsLrng/ call_SnsrOffsLrngRstHwTq/Subsystem5 ==

== system SF051A_SnsrOffsLrng/ call_SnsrOffsLrngRstYawAndAg/Subsystem5 ==

== system SF051A_SnsrOffsLrng/ call_SnsrOffsLrngSetHwAgOffs/Subsystem5 ==

== system SF051A_SnsrOffsLrng/ call_SnsrOffsLrngSetHwTqOffs/Subsystem5 ==

== system SF051A_SnsrOffsLrng/ call_SnsrOffsLrngSetYawRateOffs/Subsystem5 ==

== system SF051A_SnsrOffsLrng/SnsrOffsLrng/GetHwAgOffs ==
  note: Read the value in NVM
  function : TriggerPort  TriggerType=function-call
  Data Store Read1 : DataStoreRead  DataStoreName=HwAgLrngStRst
  FixdToFloat_f32_s16 : FixdToFloat/FixdToFloat_f32_s16  Param1=10
  NVM Ram : DataStoreRead  DataStoreName=SnsrOffsLrnd  DataStoreElements=SnsrOffsLrnd.HwAgOffs
  Subsystem5 : Subsystem  Description=|  mask(Copyright Information){none=on}
      | Copyright info block.                                               
      |                                                                     
      | Place copyright information at the top of every subsystem in design.
      mask prompts: none "No parameters"
      mask help: Place copyright information at the top of every subsystem in design.
      mask Display:
      | NxtrConf = 'Nexteer Confidential';
      | 
      | sys = bdroot; %handle for the current model ("system")
      | first = get_param(sys,'Created');
      | first = first(end-3:end);  %year is last four digits
      | 
      | last = get_param(sys,'LastModifiedDate');
      | if isempty(last)
      |     last = datestr(now,'yyyy');
      | else
      |     last = last(end-3:end);
      | end
      | 
      | if strcmp(first,last)
      |     fprintf('%s -- Copyright %s Nexteer',NxtrConf,first)
      | else
      |     fprintf('%s -- %s%s- %s Nexteer',NxtrConf,char(169),first,last)
      | end
  HwAgOffs_ArgOut : Outport
  HwAgLrngStRst_ArgOut : Outport  Port=2
  wires:
  NVM Ram/1 -> FixdToFloat_f32_s16/1
  FixdToFloat_f32_s16/1 -> HwAgOffs_ArgOut/1
  Data Store Read1/1 -> HwAgLrngStRst_ArgOut/1

== system SF051A_SnsrOffsLrng/SnsrOffsLrng/GetHwTqOffs ==
  note: Read the value in NVM
  function : TriggerPort  TriggerType=function-call
  Data Store Read1 : DataStoreRead  DataStoreName=HwTqLrngStRst
  FixdToFloat_f32_s16 : FixdToFloat/FixdToFloat_f32_s16  Param1=12
  NVM Ram : DataStoreRead  DataStoreName=SnsrOffsLrnd  DataStoreElements=SnsrOffsLrnd.HwTqOffs
  Subsystem5 : Subsystem  Description=|  mask(Copyright Information){none=on}
      | Copyright info block.                                               
      |                                                                     
      | Place copyright information at the top of every subsystem in design.
      mask prompts: none "No parameters"
      mask help: Place copyright information at the top of every subsystem in design.
      mask Display:
      | NxtrConf = 'Nexteer Confidential';
      | 
      | sys = bdroot; %handle for the current model ("system")
      | first = get_param(sys,'Created');
      | first = first(end-3:end);  %year is last four digits
      | 
      | last = get_param(sys,'LastModifiedDate');
      | if isempty(last)
      |     last = datestr(now,'yyyy');
      | else
      |     last = last(end-3:end);
      | end
      | 
      | if strcmp(first,last)
      |     fprintf('%s -- Copyright %s Nexteer',NxtrConf,first)
      | else
      |     fprintf('%s -- %s%s- %s Nexteer',NxtrConf,char(169),first,last)
      | end
  HwTqOffs_ArgOut : Outport
  HwTqLrngStRst_ArgOut : Outport  Port=2
  wires:
  FixdToFloat_f32_s16/1 -> HwTqOffs_ArgOut/1
  NVM Ram/1 -> FixdToFloat_f32_s16/1
  Data Store Read1/1 -> HwTqLrngStRst_ArgOut/1

== system SF051A_SnsrOffsLrng/SnsrOffsLrng/GetYawRateOffs ==
  note: Read the value in NVM
  function : TriggerPort  TriggerType=function-call
  Data Store Read1 : DataStoreRead  DataStoreName=VehYawRateLrngStRst
  FixdToFloat_f32_s16 : FixdToFloat/FixdToFloat_f32_s16  Param1=9
  NVM Ram : DataStoreRead  DataStoreName=SnsrOffsLrnd  DataStoreElements=SnsrOffsLrnd.YawRateOffs
  Subsystem5 : Subsystem  Description=|  mask(Copyright Information){none=on}
      | Copyright info block.                                               
      |                                                                     
      | Place copyright information at the top of every subsystem in design.
      mask prompts: none "No parameters"
      mask help: Place copyright information at the top of every subsystem in design.
      mask Display:
      | NxtrConf = 'Nexteer Confidential';
      | 
      | sys = bdroot; %handle for the current model ("system")
      | first = get_param(sys,'Created');
      | first = first(end-3:end);  %year is last four digits
      | 
      | last = get_param(sys,'LastModifiedDate');
      | if isempty(last)
      |     last = datestr(now,'yyyy');
      | else
      |     last = last(end-3:end);
      | end
      | 
      | if strcmp(first,last)
      |     fprintf('%s -- Copyright %s Nexteer',NxtrConf,first)
      | else
      |     fprintf('%s -- %s%s- %s Nexteer',NxtrConf,char(169),first,last)
      | end
  VehYawRateOffs_ArgOut : Outport
  VehYawRateLrngStRst_ArgOut : Outport  Port=2
  wires:
  NVM Ram/1 -> FixdToFloat_f32_s16/1
  FixdToFloat_f32_s16/1 -> VehYawRateOffs_ArgOut/1
  Data Store Read1/1 -> VehYawRateLrngStRst_ArgOut/1

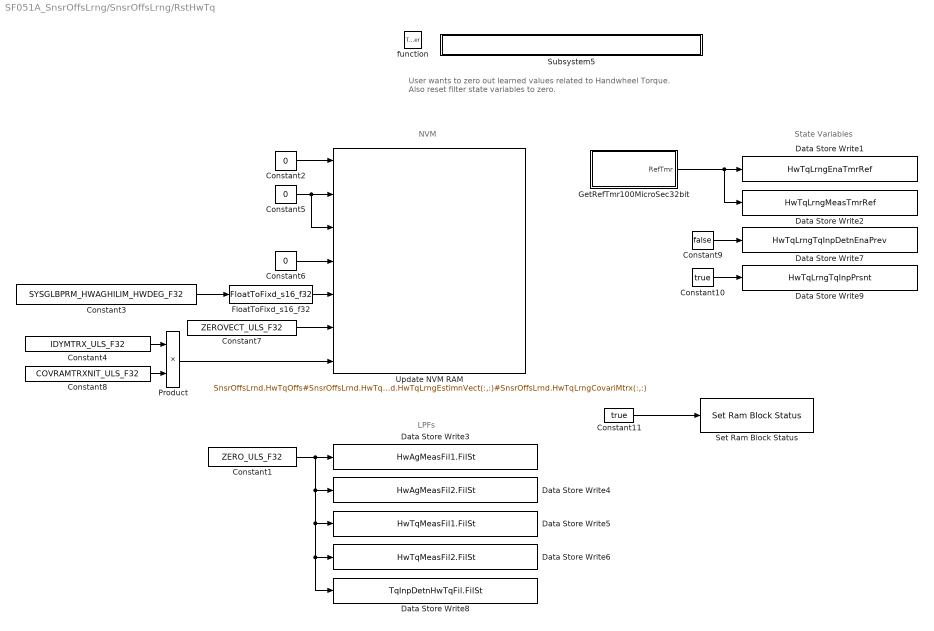
== system SF051A_SnsrOffsLrng/SnsrOffsLrng/RstHwTq ==
  note: LPFs
  note: State Variables
  note: NVM
  note: User wants to zero out learned values related to Handwheel Torque.
      | Also reset filter state variables to zero.
  function : TriggerPort  TriggerType=function-call
  Constant1 : Constant  Value=ZERO_ULS_F32  OutDataTypeStr=single
      settings: AttributesFormatString=%<OutDataTypeStr>
  Constant10 : Constant  Value=true  OutDataTypeStr=boolean
      settings: AttributesFormatString=%<OutDataTypeStr>
  Constant11 : Constant  Value=true  OutDataTypeStr=boolean
      settings: AttributesFormatString=%<OutDataTypeStr>
  Constant2 : Constant  Value=0  OutDataTypeStr=int16
      settings: AttributesFormatString=%<OutDataTypeStr>
  Constant3 : Constant  Value=SYSGLBPRM_HWAGHILIM_HWDEG_F32  OutDataTypeStr=single
      settings: AttributesFormatString=%<OutDataTypeStr>
  Constant4 : Constant  Value=IDYMTRX_ULS_F32  VectorParams1D=off  OutDataTypeStr=single
      settings: AttributesFormatString=%<OutDataTypeStr>, 3x3
  Constant5 : Constant  Value=0  OutDataTypeStr=uint16
      settings: AttributesFormatString=%<OutDataTypeStr>
  Constant6 : Constant  Value=0  OutDataTypeStr=uint8
      settings: AttributesFormatString=%<OutDataTypeStr>
  Constant7 : Constant  Value=ZEROVECT_ULS_F32  VectorParams1D=off  OutDataTypeStr=single
      settings: AttributesFormatString=%<OutDataTypeStr>, 3x1
  Constant8 : Constant  Value=COVRAMTRXNIT_ULS_F32  OutDataTypeStr=single
      settings: AttributesFormatString=%<OutDataTypeStr>
  Constant9 : Constant  Value=false  OutDataTypeStr=boolean
      settings: AttributesFormatString=%<OutDataTypeStr>
  Data Store Write1 : DataStoreWrite  DataStoreName=HwTqLrngEnaTmrRef
  Data Store Write2 : DataStoreWrite  DataStoreName=HwTqLrngMeasTmrRef
  Data Store Write3 : DataStoreWrite  DataStoreName=HwAgMeasFil1  DataStoreElements=HwAgMeasFil1.FilSt
  Data Store Write4 : DataStoreWrite  DataStoreName=HwAgMeasFil2  DataStoreElements=HwAgMeasFil2.FilSt
  Data Store Write5 : DataStoreWrite  DataStoreName=HwTqMeasFil1  DataStoreElements=HwTqMeasFil1.FilSt
  Data Store Write6 : DataStoreWrite  DataStoreName=HwTqMeasFil2  DataStoreElements=HwTqMeasFil2.FilSt
  Data Store Write7 : DataStoreWrite  DataStoreName=HwTqLrngTqInpDetnEnaPrev
  Data Store Write8 : DataStoreWrite  DataStoreName=TqInpDetnHwTqFil  DataStoreElements=TqInpDetnHwTqFil.FilSt
  Data Store Write9 : DataStoreWrite  DataStoreName=HwTqLrngTqInpPrsnt
  FloatToFixd_s16_f32 : FloatToFixd/FloatToFixd_s16_f32  Param1=4
  GetRefTmr100MicroSec32bit : Subsystem
  Product : Product
  Set Ram Block Status : NxtrNvM/Set Ram Block Status  FuncName=Set Ram Block Status  NvMBlockName=SnsrOffsLrnd  VoidFuncRtn=on  BlockChanged_DSN=NvMSRBS_BlockChanged7  Return_DSN=NvMSRBS_Return7
      settings: AttributesFormatString=%<FuncName>
  Subsystem5 : Subsystem  Description=|  mask(Copyright Information){none=on}
      | Copyright info block.                                               
      |                                                                     
      | Place copyright information at the top of every subsystem in design.
      mask prompts: none "No parameters"
      mask help: Place copyright information at the top of every subsystem in design.
      mask Display:
      | NxtrConf = 'Nexteer Confidential';
      | 
      | sys = bdroot; %handle for the current model ("system")
      | first = get_param(sys,'Created');
      | first = first(end-3:end);  %year is last four digits
      | 
      | last = get_param(sys,'LastModifiedDate');
      | if isempty(last)
      |     last = datestr(now,'yyyy');
      | else
      |     last = last(end-3:end);
      | end
      | 
      | if strcmp(first,last)
      |     fprintf('%s -- Copyright %s Nexteer',NxtrConf,first)
      | else
      |     fprintf('%s -- %s%s- %s Nexteer',NxtrConf,char(169),first,last)
      | end
  Update NVM RAM : DataStoreWrite  DataStoreName=SnsrOffsLrnd  DataStoreElements=SnsrOffsLrnd.HwTqOffs#SnsrOffsLrnd.HwTqLrngSampleCntNeg#SnsrOffsLrnd.HwTqLrngSampleCntPos#SnsrOffsLrnd.HwTqLrngSts#SnsrOffsLrnd.HwTqLrngHwAgRef#SnsrOffsLrnd.HwTqLrngEstimnVect(:,:)#SnsrOffsLrnd.HwTqLrngCovariMtrx(:,:)
  wires:
  Constant2/1 -> Update NVM RAM/1
  Constant1/1 -> Data Store Write8/1, Data Store Write6/1, Data Store Write5/1, Data Store Write4/1, Data Store Write3/1
  GetRefTmr100MicroSec32bit/1(RefTmr) -> Data Store Write2/1, Data Store Write1/1
  Constant3/1 -> FloatToFixd_s16_f32/1
  Constant5/1 -> Update NVM RAM/3, Update NVM RAM/2
  Constant6/1 -> Update NVM RAM/4
  Constant7/1 -> Update NVM RAM/6
  Constant4/1 -> Product/1
  Constant8/1 -> Product/2
  Product/1 -> Update NVM RAM/7
  Constant9/1 -> Data Store Write7/1
  Constant10/1 -> Data Store Write9/1
  FloatToFixd_s16_f32/1 -> Update NVM RAM/5
  Constant11/1 -> Set Ram Block Status/1

== system SF051A_SnsrOffsLrng/SnsrOffsLrng/RstYawAndAg ==
  note: User wants to zero out learned values related to Yaw Rate and Handwheel Angle.
      | Also reset filter state variables to zero.
  note: To write the same than it is written as YawRateOffs
  note: POC
  note: YOC
  function : TriggerPort  TriggerType=function-call
  Constant1 : Constant  Value=ZERO_ULS_F32  OutDataTypeStr=single
      settings: AttributesFormatString=%<OutDataTypeStr>
  Constant10 : Constant  Value=true  OutDataTypeStr=boolean
      settings: AttributesFormatString=%<OutDataTypeStr>
  Constant{2,4,7..8,11} (5 alike) : Constant  Value=0  OutDataTypeStr=int16
      settings: AttributesFormatString=%<OutDataTypeStr>
  Constant14 : Constant  Value=ZERO_ULS_F32  OutDataTypeStr=single
  Constant3 : Constant  Value=false  OutDataTypeStr=boolean
      settings: AttributesFormatString=%<OutDataTypeStr>
  Constant5 : Constant  Value=YAWELPDTIHILIM_MINS_F32  OutDataTypeStr=single
  Data Store Write1 : DataStoreWrite  DataStoreName=HwAgLrngFil1  DataStoreElements=HwAgLrngFil1.FilSt
  Data Store Write2 : DataStoreWrite  DataStoreName=YawLrngFil2  DataStoreElements=YawLrngFil2.FilSt
  Data Store Write3 : DataStoreWrite  DataStoreName=HwAgLrngFil2  DataStoreElements=HwAgLrngFil2.FilSt
  Data Store Write4 : DataStoreWrite  DataStoreName=YawLrngFil1  DataStoreElements=YawLrngFil1.FilSt
  Data Store Write5 : DataStoreWrite  DataStoreName=HwAgLrngSysTqFil1  DataStoreElements=HwAgLrngSysTqFil1.FilSt
  Data Store Write6 : DataStoreWrite  DataStoreName=YawLrngElpdLrngTi
  Data Store Write7 : DataStoreWrite  DataStoreName=HwAgLrngSysTqFil1  DataStoreElements=HwAgLrngSysTqFil1.FilSt
  Set Ram Block Status : NxtrNvM/Set Ram Block Status  FuncName=Set Ram Block Status  NvMBlockName=SnsrOffsLrnd  VoidFuncRtn=on  BlockChanged_DSN=NvMSRBS_BlockChanged6  Return_DSN=NvMSRBS_Return6
      settings: AttributesFormatString=%<FuncName>
  Subsystem5 : Subsystem  Description=|  mask(Copyright Information){none=on}
      | Copyright info block.                                               
      |                                                                     
      | Place copyright information at the top of every subsystem in design.
      mask prompts: none "No parameters"
      mask help: Place copyright information at the top of every subsystem in design.
      mask Display:
      | NxtrConf = 'Nexteer Confidential';
      | 
      | sys = bdroot; %handle for the current model ("system")
      | first = get_param(sys,'Created');
      | first = first(end-3:end);  %year is last four digits
      | 
      | last = get_param(sys,'LastModifiedDate');
      | if isempty(last)
      |     last = datestr(now,'yyyy');
      | else
      |     last = last(end-3:end);
      | end
      | 
      | if strcmp(first,last)
      |     fprintf('%s -- Copyright %s Nexteer',NxtrConf,first)
      | else
      |     fprintf('%s -- %s%s- %s Nexteer',NxtrConf,char(169),first,last)
      | end
  Update NVM RAM : DataStoreWrite  DataStoreName=SnsrOffsLrnd  DataStoreElements=SnsrOffsLrnd.YawRateOffs#SnsrOffsLrnd.YawRateOffsVld#SnsrOffsLrnd.YawRateElpdTi
  Update NVM RAM1 : DataStoreWrite  DataStoreName=SnsrOffsLrnd  DataStoreElements=SnsrOffsLrnd.HwAgOffs#SnsrOffsLrnd.HwAgLrndTi#SnsrOffsLrnd.HwAgLrngHwAgFilSt#SnsrOffsLrnd.HwAgLrngSysTqFilSt#SnsrOffsLrnd.HwAgLrngYawOffsRef
  wires:
  Constant2/1 -> Update NVM RAM/1
  Constant3/1 -> Update NVM RAM/2
  Constant5/1 -> Update NVM RAM/3
  Constant14/1 -> Update NVM RAM1/2
  Constant4/1 -> Update NVM RAM1/1
  Constant7/1 -> Update NVM RAM1/3
  Constant8/1 -> Update NVM RAM1/4
  Constant10/1 -> Set Ram Block Status/1
  Constant11/1 -> Update NVM RAM1/5
  Constant1/1 -> Data Store Write4/1, Data Store Write2/1, Data Store Write1/1, Data Store Write3/1, Data Store Write5/1, Data Store Write7/1, Data Store Write6/1
